simulink subsystem "Trajectory"  (R2020a)
settings: Solver=VariableStepAuto  StartTime=0.0  StopTime=10.0  RelTol=1e-3
values from neighbouring files (symbols this model uses):
  Ts = 0.1    [main_adaptive_mpc.m]    (also in matlab.mat; newNewTraj.m = 0.25; plant_init.m)
libraries: aerolibutil x2
settings Model: Creator=Lamarre  LastModifiedBy=lamarre

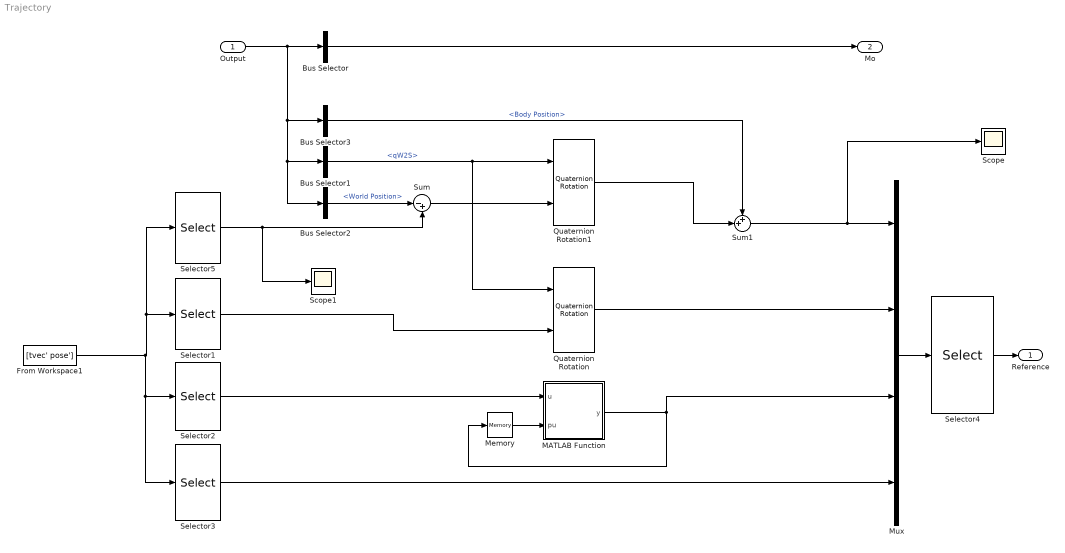
== system Trajectory ==
  Output : Inport
  Bus Selector : BusSelector  OutputSignals=Body Position,Roll;Pitch; Yaw,Body Velocity,Angular Rate  OutputAsBus=on
  Bus Selector1 : BusSelector  OutputSignals=qW2S
  Bus Selector2 : BusSelector  OutputSignals=World Position
  Bus Selector3 : BusSelector  OutputSignals=Body Position
  From Workspace1 : FromWorkspace  VariableName=[tvec' pose']  SampleTime=Ts  Interpolate=off  OutputAfterFinalValue=Holding final value
  MATLAB Function : MATLAB Function  TreatAsAtomicUnit=on  SystemSampleTime=Ts
  Memory : Memory
  Mux : Mux
  Quaternion Rotation : aerolibutil/Quaternion Rotation
  Quaternion Rotation1 : aerolibutil/Quaternion Rotation
  Scope : Scope
  Scope1 : Scope
  Selector1 : Selector  InputPortWidth=12  IndexOptions=Index vector (dialog)  Indices=[7:9]  OutputSizes=1
  Selector2 : Selector  InputPortWidth=12  IndexOptions=Index vector (dialog)  Indices=[4:6]  OutputSizes=1
  Selector3 : Selector  InputPortWidth=12  IndexOptions=Index vector (dialog)  Indices=[10:12]  OutputSizes=1
  Selector4 : Selector  InputPortWidth=12  IndexOptions=Index vector (dialog)  Indices=[1:3,7:9,4:6,10:12]  OutputSizes=1
  Selector5 : Selector  InputPortWidth=12  IndexOptions=Index vector (dialog)  Indices=[1:3]  OutputSizes=1
  Sum : Sum  Inputs=|-+
  Sum1 : Sum  Inputs=++|
  Reference : Outport
  Mo : Outport  Port=2
  wires:
  Quaternion Rotation/1 -> Mux/2
  Memory/1 -> MATLAB Function/2(pu)
  Selector1/1 -> Quaternion Rotation/2
  MATLAB Function/1(y) -> Mux/3, Memory/1
  Mux/1 -> Selector4/1
  Selector3/1 -> Mux/4
  Output/1 -> Bus Selector2/1, Bus Selector1/1, Bus Selector3/1, Bus Selector/1
  Bus Selector2/1 -> Sum/1  "<World Position>"
  Selector4/1 -> Reference/1
  Sum1/1 -> Mux/1, Scope/1
  Bus Selector/1 -> Mo/1
  Quaternion Rotation1/1 -> Sum1/2
  Bus Selector1/1 -> Quaternion Rotation/1, Quaternion Rotation1/1  "<qW2S>"
  Sum/1 -> Quaternion Rotation1/2
  Selector5/1 -> Sum/2, Scope1/1
  Bus Selector3/1 -> Sum1/1  "<Body Position>"
  Selector2/1 -> MATLAB Function/1(u)
  From Workspace1/1 -> Selector3/1, Selector2/1, Selector5/1, Selector1/1

== matlab function Trajectory/MATLAB Function ==
  data: u input; y output; pu input
function y = fcn(u,pu)
y=u;
if abs(pu(3)-u(3))>pi   
 y(3)=(pi+u(3))+pi;   
end
